simulink model "train_anarx"  (R2019a)
settings: Solver=FixedStepAuto  StartTime=0.0  StopTime=10.0  FixedStep=2.5e-4  RelTol=1e-3  EnableMultiTasking=on
PostLoadFcn:
  | , if any(exist('dsrtsu_mdlpostloadfcn', 'file') == [2, 3, 6]), try dsrtsu_mdlpostloadfcn('Execute', bdroot); catch fprintf('Error in PostLoadFcn (dsrtsu_mdlpostloadfcn) for model "%s":\n %s\n', bdroot, lasterr); end, end,
InitFcn:
  | Sicherheitssysteme_INIT
values from neighbouring files (symbols this model uses):
  duration = 1    [Sicherheitssysteme_INIT.m]
  MOTOREN_ANZAHL = numel(zero_poses)    [Sicherheitssysteme_INIT.m]
  R = (upper-lower).*rand(1, n) + lower    [Sicherheitssysteme_INIT.m]
  SAMPLE_TIME = 0.0002    [Sicherheitssysteme_INIT.m]
  T = 0.1    [Sicherheitssysteme_INIT.m]
  WS_MAX_LENGTHS = [-0.1]    [Sicherheitssysteme_INIT.m]
  WS_MAX_VEL_m_s = 0.4    [Sicherheitssysteme_INIT.m]
  WS_MIN_LENGTHS = [-0.2]    [Sicherheitssysteme_INIT.m]
  zero_poses = [     3143153400]    [Sicherheitssysteme_INIT.m]
libraries: simulink x1
PreSaveFcn:
  | , if any(exist('dsmpb_private', 'file') == [2, 3, 6]), try, dsmpb_private('dsmpb_mdlclblib', 'PreSave', bdroot); catch, disp(lasterr); end, end,
CloseFcn:
  | , if any(exist('dsmpb_private', 'file') == [2, 3, 6]), try, dsmpb_private('dsmpb_mdlclblib', 'Close', bdroot); catch, disp(lasterr); end, end,
settings Model: DSMPB_DATASERVER_ModelPortLibVersion1=8  DSMPB_DATASERVER_DataServerVersion1=6  DSMPB_DATASERVER_DataServerStreamVersion1=3  Creator=CableRobot  LastModifiedBy=brandlju
settings DataIOCC: ReturnWorkspaceOutputs=off
settings OptimizationCC: LocalBlockOutputs=off
settings DebuggingCC: SFUnexpectedBacktrackingDiag=warning  SFNoUnconditionalDefaultTransitionDiag=warning  ArithmeticOperatorsInVariantConditions=warning
settings SFSimCC: SimUseLocalCustomCode=off
settings RTWCC: SystemTargetFile=TwinCAT.tlc  GenCodeOnly=on  MakeCommand=make_tct  TemplateMakefile=tct_msbuild.tmf  Description=TwinCAT Target  GenerateReport=on  RTWUseLocalCustomCode=off  TargetLang=C++
settings CodeAppCC: StateflowObjectComments=on
settings STFCustomTargetCC: TargetLangStandard=C++03 (ISO)  CompOptLevelCompliant=on  MATLABClassNameForMDSCustomization=Simulink.SoftwareTarget.TargetSpecificTriggerConfigurationBase  SystemTargetFile=TwinCAT.tlc
settings ConfigComp: CovMetricSettings=dw  CovHtmlReporting=on  CovSaveCumulativeToWorkspaceVar=on  CovSaveSingleToWorkspaceVar=on  CovExternalEMLEnable=off

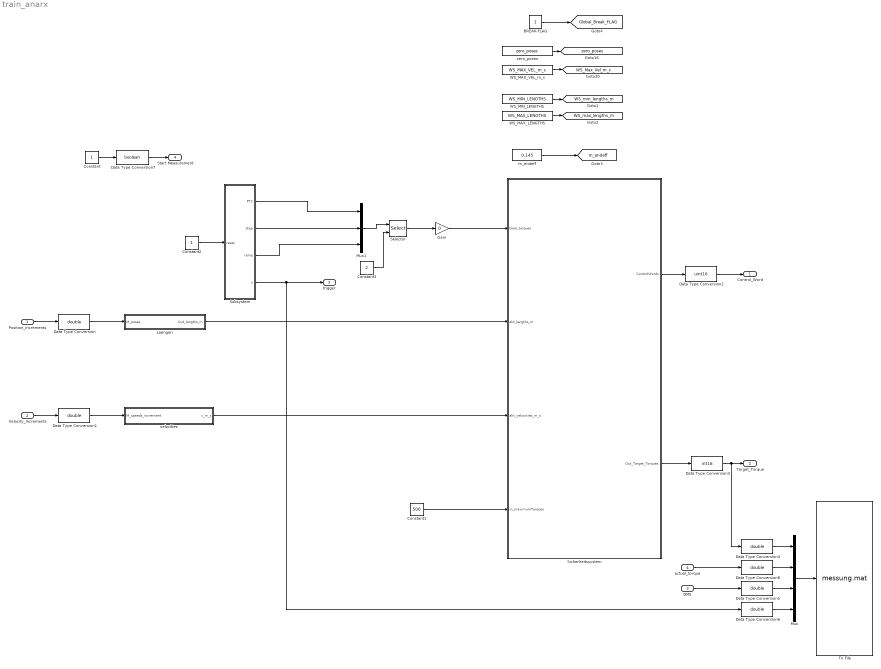
== system train_anarx ==
  Position_Increments : Inport  OutDataTypeStr=uint32
  Velocity_Increments : Inport  Port=2
  DMS : Inport  Port=3  OutDataTypeStr=int32
  actual_torque : Inport  Port=4  OutDataTypeStr=int16
  BREAK-FLAG : Constant
  Constant : Constant
  Constant1 : Constant  Value=500
  Constant2 : Constant
  Constant3 : Constant  Value=2
  Data Type Conversion{,1,4..6,8} (6 alike) : DataTypeConversion  OutDataTypeStr=double
  Data Type Conversion2 : DataTypeConversion  OutDataTypeStr=uint16
  Data Type Conversion3 : DataTypeConversion  OutDataTypeStr=int16
  Data Type Conversion7 : DataTypeConversion  OutDataTypeStr=boolean
  Gain : Gain  Gain=0
  Laengen : Subsystem
  Mux : Mux
  Mux1 : Mux  Inputs=3
  Selector : Selector  InputPortWidth=3  IndexOptions=Index vector (port)  Indices=[1 3]  OutputSizes=1
  Sicherheitssystem : Subsystem
  Subsystem : Subsystem
  To File : ToFile  Filename=messung.mat  MatrixName=data
  WS_MAX_LENGTHS : Constant  Value=WS_MAX_LENGTHS
  WS_MAX_VEL_m_s : Constant  Value=WS_MAX_VEL_m_s
  WS_MIN_LENGTHS : Constant  Value=WS_MIN_LENGTHS
  m_endeff : Constant  Value=0.145
  velocities : MATLAB Function  TreatAsAtomicUnit=on
  zero_poses : Constant  Value=zero_poses
  Control_Word : Outport  OutDataTypeStr=uint16
  Target_Torque : Outport  Port=2  OutDataTypeStr=int16
  trigger : Outport  Port=3  VectorParamsAs1DForOutWhenUnconnected=on
  Start Measurement : Outport  Port=4  OutDataTypeStr=boolean
  tag scope: Global_Break_FLAG=global, WS_Max_Vel_m_s=global, WS_max_lengths_m=global, WS_min_lengths_m=global, m_endeff=global, zero_poses=global
  wires:
  m_endeff/1 -> [m_endeff]
  WS_MAX_VEL_m_s/1 -> [WS_Max_Vel_m_s]
  WS_MIN_LENGTHS/1 -> [WS_min_lengths_m]
  WS_MAX_LENGTHS/1 -> [WS_max_lengths_m]
  Laengen/1(Out_lengths_m) -> Sicherheitssystem/2(akt_lengths_m)
  velocities/1(v_m_s) -> Sicherheitssystem/3(akt_velocities_m_s)
  BREAK-FLAG/1 -> [Global_Break_FLAG]
  zero_poses/1 -> [zero_poses]
  Constant1/1 -> Sicherheitssystem/4(in_maximumTorques)
  Position_Increments/1 -> Data Type Conversion/1
  Velocity_Increments/1 -> Data Type Conversion1/1
  Sicherheitssystem/1(ControlWords) -> Data Type Conversion2/1
  Sicherheitssystem/2(Out_Target_Torques) -> Data Type Conversion3/1
  Data Type Conversion/1 -> Laengen/1(M_poses)
  Data Type Conversion1/1 -> velocities/1(M_speeds_increment)
  Data Type Conversion2/1 -> Control_Word/1
  Subsystem/3(ramp) -> Mux1/3
  Subsystem/1(PT2) -> Mux1/1
  Data Type Conversion4/1 -> Mux/1
  Data Type Conversion3/1 -> Data Type Conversion4/1, Target_Torque/1
  Subsystem/4(y) -> Data Type Conversion6/1, trigger/1
  Mux/1 -> To File/1
  Data Type Conversion5/1 -> Mux/3
  Subsystem/2(step) -> Mux1/2
  Data Type Conversion6/1 -> Mux/4
  Constant/1 -> Data Type Conversion7/1
  Data Type Conversion7/1 -> Start Measurement/1
  DMS/1 -> Data Type Conversion5/1
  Gain/1 -> Sicherheitssystem/1(Goal_torques)
  Constant2/1 -> Subsystem/1(reset)
  Data Type Conversion8/1 -> Mux/2
  actual_torque/1 -> Data Type Conversion8/1
  Mux1/1 -> Selector/1
  Selector/1 -> Gain/1
  Constant3/1 -> Selector/2

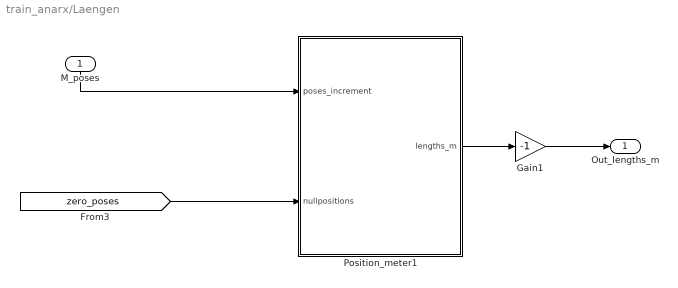
== system train_anarx/Laengen ==
  M_poses : Inport
  Gain1 : Gain  Gain=-1
  Position_meter1 : MATLAB Function  TreatAsAtomicUnit=on
  Out_lengths_m : Outport
  wires:
  Position_meter1/1(lengths_m) -> Gain1/1
  M_poses/1 -> Position_meter1/1(poses_increment)
  Gain1/1 -> Out_lengths_m/1
  [zero_poses] -> Position_meter1/2(nullpositions)

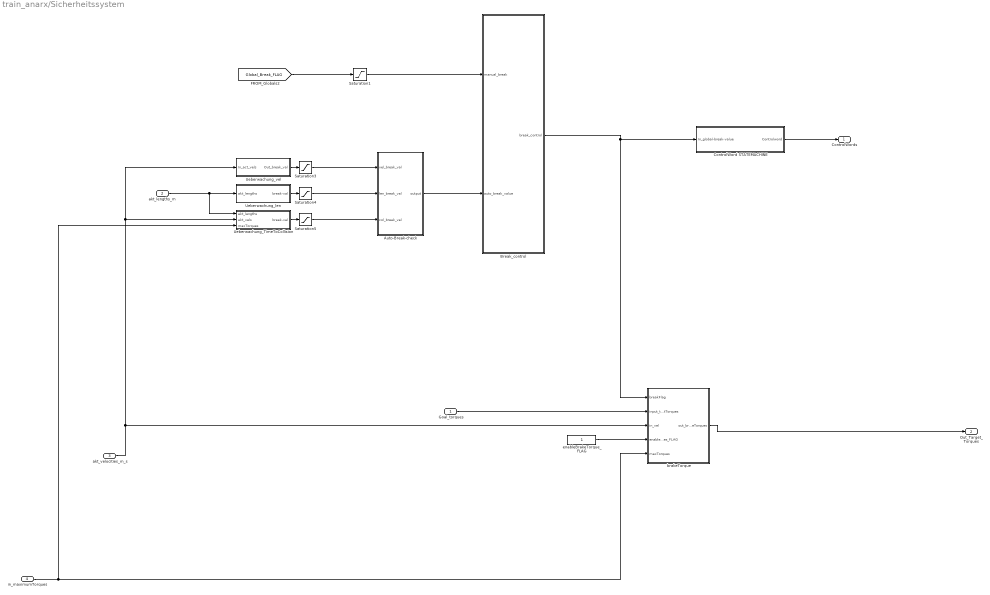
== system train_anarx/Sicherheitssystem ==
  Goal_torques : Inport
  akt_lengths_m : Inport  Port=2
  akt_velocities_m_s : Inport  Port=3
  in_maximumTorques : Inport  Port=4
  Auto-Break-check : MATLAB Function  TreatAsAtomicUnit=on
  Break_control : MATLAB Function  TreatAsAtomicUnit=on
  ControlWord STATEMACHINE : Subsystem
  Saturation1 : Saturate  UpperLimit=1  LowerLimit=0
  Saturation3 : Saturate  UpperLimit=inf  LowerLimit=0
  Saturation4 : Saturate  UpperLimit=inf  LowerLimit=0
  Saturation5 : Saturate  UpperLimit=inf  LowerLimit=0
  Ueberwachung_TimeToCollision : Subsystem
  Ueberwachung_len : Subsystem
  Ueberwachung_vel : Subsystem
  brakeTorque : MATLAB Function  TreatAsAtomicUnit=on
  enableBrakeTorque_FLAG : Constant
  ControlWords : Outport
  Out_Target_Torques : Outport  Port=2
  wires:
  ControlWord STATEMACHINE/1(Controlword) -> ControlWords/1
  [Global_Break_FLAG] -> Saturation1/1
  Break_control/1(break_control) -> brakeTorque/1(breakFlag), ControlWord STATEMACHINE/1(In_global-break-value)
  Auto-Break-check/1(output) -> Break_control/2(auto_break_value)
  Saturation1/1 -> Break_control/1(manual_break)
  akt_velocities_m_s/1 -> brakeTorque/3(in_vel), Ueberwachung_TimeToCollision/2(akt_vels), Ueberwachung_vel/1(In_act_vels)
  Ueberwachung_vel/1(Out_break_val) -> Saturation3/1
  Saturation3/1 -> Auto-Break-check/1(vel_break_val)
  akt_lengths_m/1 -> Ueberwachung_TimeToCollision/1(akt_lengths), Ueberwachung_len/1(akt_lengths)
  Ueberwachung_len/1(break-val) -> Saturation4/1
  Saturation4/1 -> Auto-Break-check/2(len_break_val)
  brakeTorque/1(out_brakeTorques) -> Out_Target_Torques/1
  in_maximumTorques/1 -> Ueberwachung_TimeToCollision/3(maxTorques), brakeTorque/5(maxTorques)
  Goal_torques/1 -> brakeTorque/2(input_targetTorques)
  enableBrakeTorque_FLAG/1 -> brakeTorque/4(enableBrakeTorques_FLAG)
  Ueberwachung_TimeToCollision/1(break-val) -> Saturation5/1
  Saturation5/1 -> Auto-Break-check/3(col_break_val)

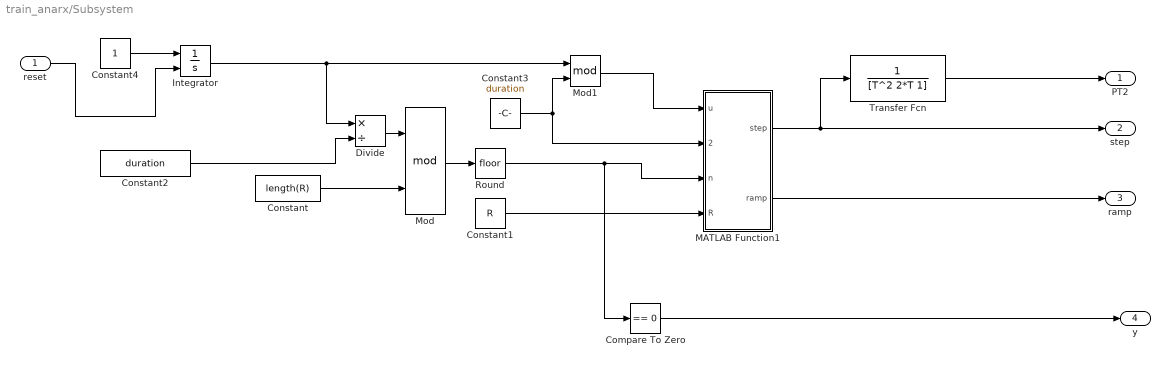
== system train_anarx/Subsystem ==
  reset : Inport
  Compare To Zero : simulink/Logic and Bit Operations/Compare To Zero  relop===  OutDataTypeStr=uint8
  Constant : Constant  Value=length(R)
  Constant1 : Constant  Value=R
  Constant2 : Constant  Value=duration
  Constant3 : Constant  Value=duration
  Constant4 : Constant
  Divide : Product  Inputs=*/
  Integrator : Integrator  ExternalReset=falling
  MATLAB Function1 : MATLAB Function  TreatAsAtomicUnit=on
  Mod : Math  Operator=mod  SaturateOnIntegerOverflow=on
  Mod1 : Math  Operator=mod  SaturateOnIntegerOverflow=on
  Round : Rounding
  Transfer Fcn : TransferFcn  Denominator=[T^2 2*T 1]
  PT2 : Outport  VectorParamsAs1DForOutWhenUnconnected=on
  step : Outport  Port=2  VectorParamsAs1DForOutWhenUnconnected=on
  ramp : Outport  Port=3  VectorParamsAs1DForOutWhenUnconnected=on
  y : Outport  Port=4  VectorParamsAs1DForOutWhenUnconnected=on
  wires:
  Constant/1 -> Mod/2
  Constant3/1 -> Mod1/2, MATLAB Function1/2(duration)
  Integrator/1 -> Divide/1, Mod1/1
  Divide/1 -> Mod/1
  Constant2/1 -> Divide/2
  Round/1 -> Compare To Zero/1, MATLAB Function1/3(n)
  Constant1/1 -> MATLAB Function1/4(R)
  MATLAB Function1/1(step) -> step/1, Transfer Fcn/1
  Mod/1 -> Round/1
  MATLAB Function1/2(ramp) -> ramp/1
  Mod1/1 -> MATLAB Function1/1(u)
  Transfer Fcn/1 -> PT2/1
  Compare To Zero/1 -> y/1
  Constant4/1 -> Integrator/1
  reset/1 -> Integrator/2

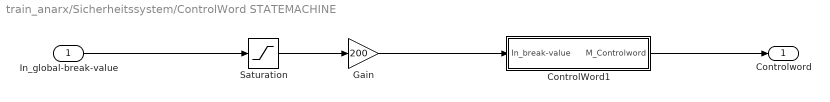
== system train_anarx/Sicherheitssystem/ControlWord STATEMACHINE ==
  In_global-break-value : Inport
  ControlWord1 : Subsystem
  Gain : Gain  Gain=200
  Saturation : Saturate  UpperLimit=1  LowerLimit=0
  Controlword : Outport
  wires:
  ControlWord1/1(M_Controlword) -> Controlword/1
  Gain/1 -> ControlWord1/1(In_break-value)
  In_global-break-value/1 -> Saturation/1
  Saturation/1 -> Gain/1

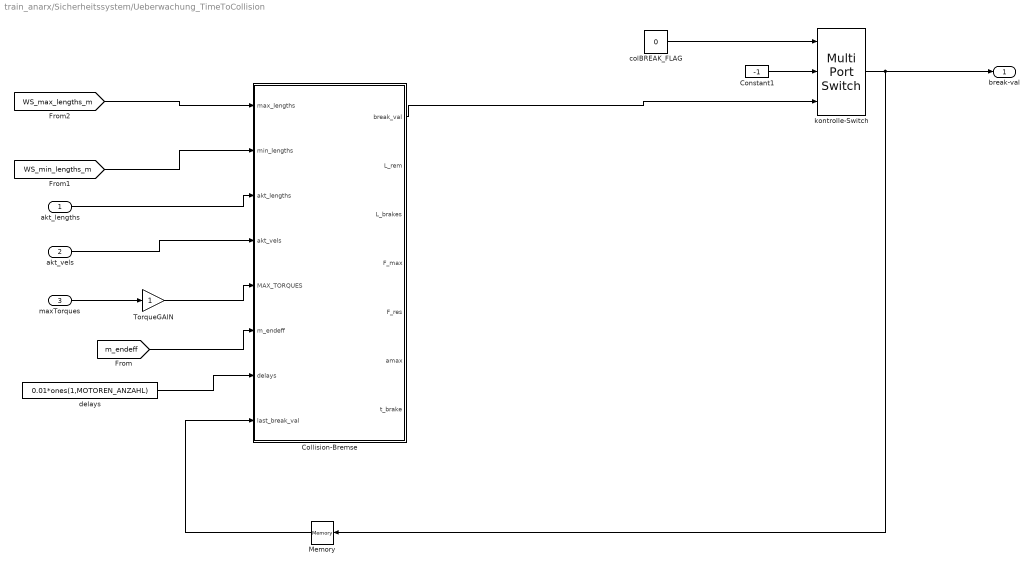
== system train_anarx/Sicherheitssystem/Ueberwachung_TimeToCollision ==
  akt_lengths : Inport
  akt_vels : Inport  Port=2
  maxTorques : Inport  Port=3
  Collision-Bremse : MATLAB Function  TreatAsAtomicUnit=on
  Constant1 : Constant  Value=-1
  Memory : Memory
  TorqueGAIN : Gain
  colBREAK_FLAG : Constant  Value=0
  delays : Constant  Value=0.01*ones(1,MOTOREN_ANZAHL)
  kontrolle-Switch : MultiPortSwitch  DataPortOrder=Zero-based contiguous  Inputs=2  zeroidx=on
  break-val : Outport
  wires:
  akt_lengths/1 -> Collision-Bremse/3(akt_lengths)
  [WS_min_lengths_m] -> Collision-Bremse/2(min_lengths)
  [WS_max_lengths_m] -> Collision-Bremse/1(max_lengths)
  colBREAK_FLAG/1 -> kontrolle-Switch/1
  Constant1/1 -> kontrolle-Switch/2
  kontrolle-Switch/1 -> Memory/1, break-val/1
  Collision-Bremse/1(break_val) -> kontrolle-Switch/3
  akt_vels/1 -> Collision-Bremse/4(akt_vels)
  maxTorques/1 -> TorqueGAIN/1
  [m_endeff] -> Collision-Bremse/6(m_endeff)
  Memory/1 -> Collision-Bremse/8(last_break_val)
  TorqueGAIN/1 -> Collision-Bremse/5(MAX_TORQUES)
  delays/1 -> Collision-Bremse/7(delays)

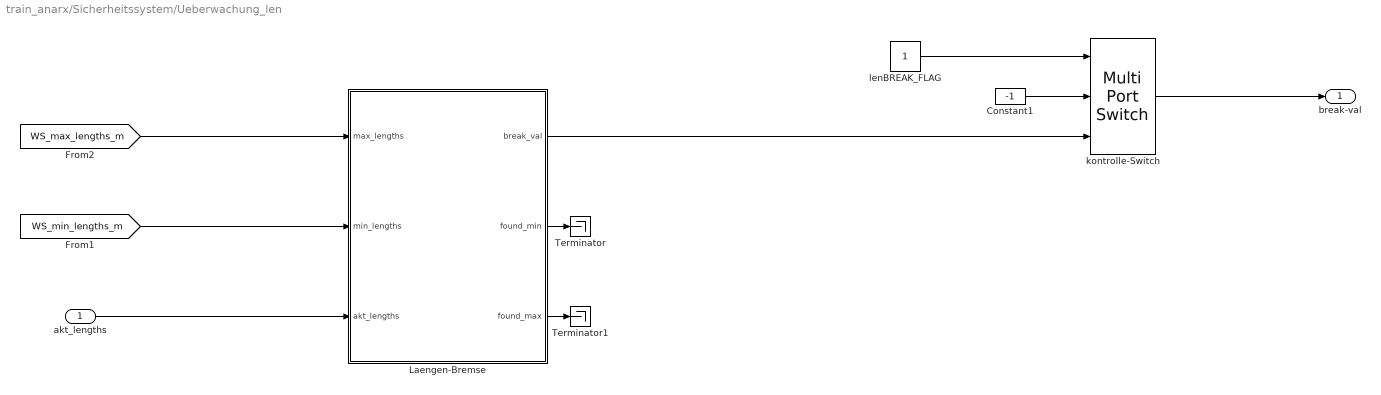
== system train_anarx/Sicherheitssystem/Ueberwachung_len ==
  akt_lengths : Inport
  Constant1 : Constant  Value=-1
  Laengen-Bremse : MATLAB Function  TreatAsAtomicUnit=on
  Terminator : Terminator
  Terminator1 : Terminator
  kontrolle-Switch : MultiPortSwitch  DataPortOrder=Zero-based contiguous  Inputs=2  zeroidx=on
  lenBREAK_FLAG : Constant
  break-val : Outport
  wires:
  Laengen-Bremse/1(break_val) -> kontrolle-Switch/3
  kontrolle-Switch/1 -> break-val/1
  Constant1/1 -> kontrolle-Switch/2
  lenBREAK_FLAG/1 -> kontrolle-Switch/1
  [WS_max_lengths_m] -> Laengen-Bremse/1(max_lengths)
  [WS_min_lengths_m] -> Laengen-Bremse/2(min_lengths)
  akt_lengths/1 -> Laengen-Bremse/3(akt_lengths)
  Laengen-Bremse/2(found_min) -> Terminator/1
  Laengen-Bremse/3(found_max) -> Terminator1/1

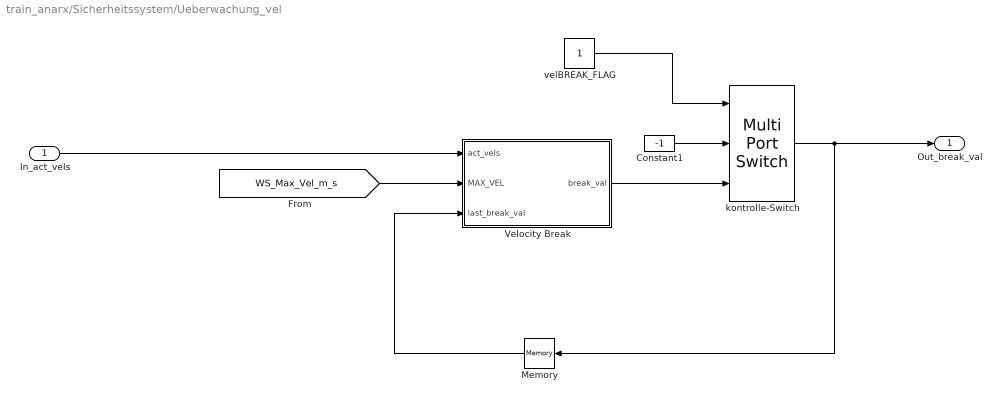
== system train_anarx/Sicherheitssystem/Ueberwachung_vel ==
  In_act_vels : Inport
  Constant1 : Constant  Value=-1
  Memory : Memory
  Velocity Break : MATLAB Function  TreatAsAtomicUnit=on
  kontrolle-Switch : MultiPortSwitch  DataPortOrder=Zero-based contiguous  Inputs=2  zeroidx=on
  velBREAK_FLAG : Constant
  Out_break_val : Outport
  wires:
  [WS_Max_Vel_m_s] -> Velocity Break/2(MAX_VEL)
  Memory/1 -> Velocity Break/3(last_break_val)
  In_act_vels/1 -> Velocity Break/1(act_vels)
  Velocity Break/1(break_val) -> kontrolle-Switch/3
  kontrolle-Switch/1 -> Out_break_val/1, Memory/1
  Constant1/1 -> kontrolle-Switch/2
  velBREAK_FLAG/1 -> kontrolle-Switch/1

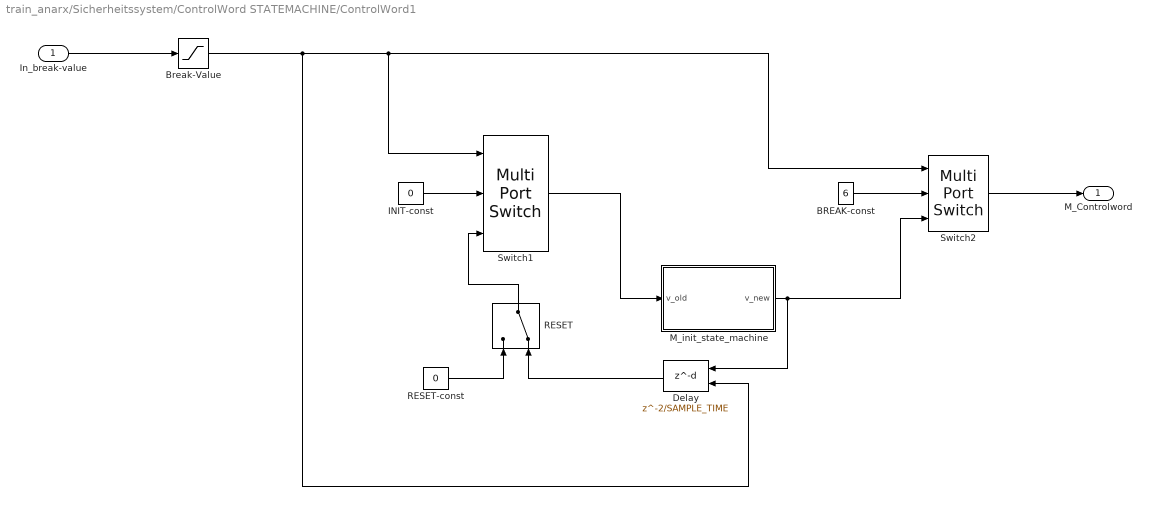
== system train_anarx/Sicherheitssystem/ControlWord STATEMACHINE/ControlWord1 ==
  In_break-value : Inport
  BREAK-const : Constant  Value=6
  Break-Value : Saturate  UpperLimit=1  LowerLimit=0
  Delay : Delay  DelayLength=2/SAMPLE_TIME  InitialCondition=0  ExternalReset=Falling
      settings: InputPortMap=u0,r5
  INIT-const : Constant  Value=0
  M_init_state_machine : MATLAB Function  TreatAsAtomicUnit=on
  RESET : ManualSwitch  CurrentSetting=0
  RESET-const : Constant  Value=0
  Switch1 : MultiPortSwitch  Inputs=2
  Switch2 : MultiPortSwitch  Inputs=2
  M_Controlword : Outport
  wires:
  M_init_state_machine/1(v_new) -> Switch2/3, Delay/1
  INIT-const/1 -> Switch1/2
  BREAK-const/1 -> Switch2/2
  Switch2/1 -> M_Controlword/1
  Delay/1 -> RESET/2
  Switch1/1 -> M_init_state_machine/1(v_old)
  RESET/1 -> Switch1/3
  RESET-const/1 -> RESET/1
  Break-Value/1 -> Switch2/1, Switch1/1, Delay/2
  In_break-value/1 -> Break-Value/1

== matlab function train_anarx/Sicherheitssystem/ControlWord STATEMACHINE/ControlWord1/M_init_state_machine ==
  data: v_new output; v_old input
function v_new = fcn(v_old)
%#codegen
%{
Die Servoklemmen der Motoren müssen gewisse Zustände durchlaufen, um in
den dauerhaften Betriebszustand zu kommen.

Diese Zustände sind in der korrekten Reihenfolge:
- Fault reset
- Shut down
- Switch on
- Enable operation

Dazu muss der Variable Controlword für jeden Zustand ein Wert übergeben
werden. Zwischen den Werten muss eine gewisse Zeit liegen. Dabei reichen
1000 Abtastschritte bei 1kHz Abtastrate des dSpace-Systems nicht aus, 2000
Abtastschritte schon. Die Werte, welche der Variable übergeben werden
lauten in der korrekten Reihenfolge:
- 0x80 (128d)
- 0x06 (  6d)
- 0x07 (  7d)
- 0x0F ( 15d)
Initial ist der Wert der Variable auf 0x00 gesetzt.
Der initale Wert sowie die Verzögerung zwischen zwei Werten kann in dem
Delay-Block editiert werden.
%}

% if (v_old ~= 15)
%     if (v_old == 0)
%         v_new = 128;
%     else if (v_old == 128)
%             v_new = 6;
%         else if (v_old == 6)
%                 v_new = 7;
%             else
%                 v_new = 15;
%             end
%         end
%     end
% else
%     v_new = 15;
% end

switch v_old
    case 128
        v_new = 6;
    case 6
        v_new = 7;
    case 7
        v_new = 15;
        
    case 15
        v_new = 15;
        
    otherwise
        v_new = 128;
end

== matlab function train_anarx/Subsystem/MATLAB Function1 ==
  data: u input; duration input; step output; n input; R input; ramp output
function [step, ramp]= fcn(u, duration, n, R)

a = mod(n, length(R))+1;
b = mod(n+1, length(R))+1;
step = R(a);

ramp = R(a)+(R(b)-R(a))*u/duration;

== matlab function train_anarx/Sicherheitssystem/Ueberwachung_vel/Velocity Break ==
  data: act_vels input; break_val output; MAX_VEL input; last_break_val input
function break_val = fcn(act_vels, MAX_VEL, last_break_val)
% Überwacht die Geschwindigkeiten aller Motoren.
%----------------------
% RETURN VALUES
% break_val:
%       0       Alle Geschwindigkeiten geringer als MAX_VEL
%     1...*     Nummer des ersten Motors der die Geschwindigkeit überschritten hat
%               (= Auslöser der Motorbremse für alle Motoren)

working_vels = abs(act_vels);

if last_break_val > 0
    break_val = last_break_val;
else
    % Motor mit zu hoher Geschwindigkeik finden
    if any(working_vels(:) >= MAX_VEL)
        break_index = find(working_vels(:) >= MAX_VEL);
        
        break_val = break_index(1);
    else
        break_val = 0;
    end
end

== matlab function train_anarx/velocities ==
  data: M_speeds_increment input; v_m_s output
function v_m_s = fcn(M_speeds_increment)

INC_TURN = 2^20;
UMFANG = 0.1 * pi;
FAKTOR = UMFANG / INC_TURN;


% Die Velocity_actual_value vom Motor ist nur 1/4 der tatsächlichen
% Geschwindigkeit... 
% (Liegt vermutlich an der Auflösung der Motoren)
temp_speed = M_speeds_increment * 4;


v_m_s = temp_speed * FAKTOR;

== matlab function train_anarx/Sicherheitssystem/Ueberwachung_len/Laengen-Bremse ==
  data: max_lengths input; min_lengths input; akt_lengths input; break_val output; found_min output; found_max output
function [break_val, found_min, found_max]= fcn(max_lengths, min_lengths, akt_lengths)
% Überwacht die Seillaengen aller Motoren.
%----------------------
% RETURN VALUES
% break_val:
%       0       Alle Seillaengen innerhalb der definierten Schranken
%     1...*     Nummer des ersten Motors der die Grenzen überschritten hat
%               (= Auslöser der Motorbremse für alle Motoren)

found_min = -1;
found_max = -1;

if any(akt_lengths > max_lengths) || any(akt_lengths < min_lengths)
    % ersten Motor mit zu überschrittenen Grenzen finden
    temp_max = find(akt_lengths > max_lengths, 1 );
    temp_min = find(akt_lengths < min_lengths, 1 );
    if isempty(temp_max) 
        temp_max = inf;
    end
    if isempty(temp_min) 
        temp_min = inf;
    end
    found_min = temp_min(1);
    found_max = temp_max(1);
    
    break_val = min( [found_min, found_max] );
    
    if all(isinf(break_val))
        break_val = NaN;
    end
    
else
    break_val = 0;
end

== matlab function train_anarx/Sicherheitssystem/Break_control ==
  data: manual_break input; auto_break_value input; break_control output
% Dieser Block ermöglicht die Freigabe, wenn der Motor noch nicht
% konfiguriert ist

% output:
% -11   manuelle Freigabe
% 1    manuelle Bremse
% 23    nicht Konfiguriert
% (24    Unterschiedliche Motorzustände)
% 25    irgend ein Motor ist im Fehlerzustand
% 26    Alle Motoren sind gesperrt
% 30    InstructionMode Error
% 99    Notaus
% 404   Fielbus Error
% sonst: automatische bremse (siehe Auto-Break-check)
%       |->  11: Workspace, 12: Laengen, 13:velocity (0:keine Bremse)

function break_control = fcn( manual_break,...
    auto_break_value)

%% "Harte" Bremsen  -  Sofort Return


% if StateDiff >= 1 % Bremse wenn nicht alle Motoren im gleichen Zustand sind
%     break_control = 24;
%     return
% end
if manual_break ~= 0 % Manuelle Bremse IMMER ausführen
    break_control = 1;
    return
end

%% "Weiche" Bremse (Systemüberwachung)
    % automatische Bremse
    break_control = auto_break_value;

== matlab function train_anarx/Sicherheitssystem/Auto-Break-check ==
  data: output output; vel_break_val input; len_break_val input; col_break_val input
function output = fcn( vel_break_val, len_break_val, col_break_val)
% gives the number of the first automatic break
%----------------------
% RETURN VALUES
% output:
%       0       keine Bremse
%       12      Längen bremse
%       13      Geschwindigkeitsbremse
%       14      Time-to-Collision


len_sum = sign( sum( len_break_val ) );
vel_sum = sign( sum( vel_break_val ) );
col_sum = sign( sum( col_break_val ) );

break_values = [len_sum; vel_sum; col_sum];


if any(break_values > 0)
    break_index = find(break_values > 0);
    output = 10 + break_index(1);
else
    output = 0;
end

== matlab function train_anarx/Sicherheitssystem/brakeTorque ==
  data: breakFlag input; input_targetTorques input; in_vel input; out_brakeTorques output; enableBrakeTorques_FLAG input; maxTorques input
function out_brakeTorques = fcn(breakFlag, input_targetTorques, in_vel, enableBrakeTorques_FLAG, maxTorques )

out_brakeTorques = ones(1, numel(input_targetTorques));


for i = 1:numel(input_targetTorques)
    out_brakeTorques(i) = input_targetTorques(i);
    
    if enableBrakeTorques_FLAG>0 && breakFlag > 0
        out_brakeTorques(i) = -sign(in_vel(i)) * maxTorques(i);
    end
    
end

== matlab function train_anarx/Sicherheitssystem/Ueberwachung_TimeToCollision/Collision-Bremse ==
  data: max_lengths input; min_lengths input; akt_lengths input; break_val output; akt_vels input; MAX_TORQUES input; m_endeff input; delays input; last_break_val input; L_rem output; L_brakes output; F_max output; F_res output; amax output; t_brake output
function [break_val, L_rem, L_brakes, F_max, F_res, amax, t_brake]= fcn(max_lengths, min_lengths, akt_lengths, akt_vels, MAX_TORQUES, m_endeff, delays, last_break_val)
% Überwacht die Seillaengen aller Motoren.
%----------------------
% RETURN VALUES
% break_val:
%       0       Alle Seillaengen innerhalb der definierten Schranken
%     1...*     Nummer des ersten Motors der die Grenzen überschritten hat
%               (= Auslöser der Motorbremse für alle Motoren)

r=0.05;
g = 9.81;

L_rem = zeros(1,numel(akt_lengths));
L_brakes = zeros(1,numel(akt_lengths));
F_max = zeros(1,numel(akt_lengths));
F_res = zeros(1,numel(akt_lengths));
amax = zeros(1,numel(akt_lengths));
t_brake = zeros(1,numel(akt_lengths));
for i = 1: numel(akt_lengths)
    if akt_vels(i) > 0
        L_rem(i) = akt_lengths(i) - min_lengths(i);
    elseif akt_vels(i) < 0
        L_rem(i) = max_lengths(i) - akt_lengths(i);
    else 
        L_rem(i) = min(akt_lengths(i) - min_lengths(i), max_lengths(i) - akt_lengths(i));
    end
    
    F_max(i) = -sign(akt_vels(i))* (MAX_TORQUES(i)/1000 /r);
    F_res(i) = max(0,F_max(i)) - m_endeff*g;
    amax(i) = abs(F_res(i))/m_endeff;
    t_brake(i) = akt_vels(i) / amax(i);
    L_brakes(i) = 0.5 * amax(i) * (t_brake(i)*t_brake(i)) + abs(akt_vels(i)*delays(i));

end


if any(L_brakes >= L_rem) 
    % ersten Motor mit zu überschrittenen Grenzen finden
    temp = find(L_brakes >= L_rem, 1 );
    break_val = temp(1);

else
    break_val = 0;
end

if last_break_val > 0
    break_val = last_break_val;
end

== matlab function train_anarx/Laengen/Position_meter1 ==
  data: poses_increment input; lengths_m output; nullpositions input
function lengths_m = fcn(poses_increment, nullpositions)
INC_TURN = 2^20;
UMFANG = 0.1 * pi;
FAKTOR = UMFANG / INC_TURN;

length_inc = poses_increment - nullpositions;
lengths_m = length_inc * FAKTOR;
